simulink model "semi_GSTA_vgain"  (R2018b)
settings: Solver=FixedStepAuto  StartTime=0.0  StopTime=30  FixedStep=0.01  RelTol=1e-3
InitFcn:
  | parameters_semi_gsta_vgain
model workspace: external: MAT-File (data not in the file)
values from neighbouring files (symbols this model uses):
  sample_time = 0.05    [parameters_semi_gsta_const.m]    (also in parameters_semi_gsta_vgain.m)
  x = [1.07906107302 2.04168763414 1.85257539652 1.93323325754 2.1580260637 1.75776173681 1.89939965925 1.8937988199 1.84120163561 1.64161458182 1.95451206586 1.46429138729 ... (9600 elements, 1600x6)]    [dat_x.mat]    (also in parameters_semi_gsta_const.m = [300   300    0.3    0.3]; parameters_semi_gsta_vgain.m = [2   2   0.05     5      1    0.3    0.3  1   0.5])
  x0 = 0.5    [parameters_semi_gsta_const.m]    (also in parameters_semi_gsta_vgain.m)
undefined symbols (not defined in the file or in its folder): v0
libraries: sdolib x1
settings Model: Creator=DING  LastModifiedBy=DNN
settings SolverCC: ZeroCrossAlgorithm=Adaptive
settings OptimizationCC: DefaultParameterBehavior=Inlined  EnhancedBackFolding=on  PassReuseOutputArgsAs=Individual arguments  MaxStackSize=64  OptimizeBlockOrder=speed  DifferentSizesBufferReuse=on
settings DebuggingCC: IgnoredZcDiagnostic=none  ParameterTunabilityLossMsg=error
settings HardwareCC: ProdBitPerPointer=32  ProdBitPerSizeT=32  ProdBitPerPtrDiffT=32  ProdLargestAtomicInteger=Long  ProdLargestAtomicFloat=Double  ProdWordSize=32  ProdHWDeviceType=ARM Compatible->ARM 11
settings SFSimCC: MATLABDynamicMemAlloc=off
settings RTWCC: SystemTargetFile=ert.tlc  TemplateMakefile=ert_default_tmf  GenerateReport=on  Toolchain=Catkin  IncludeHyperlinkInReport=on  LaunchReport=on  GenerateTraceInfo=on  GenerateTraceReport=on  GenerateTraceReportSl=on  GenerateTraceReportSf=on  GenerateTraceReportEml=on
settings CodeAppCC: ForceParamTrailComments=on  IgnoreCustomStorageClasses=off  OperatorAnnotations=on  SimulinkDataObjDesc=on  SFDataObjDesc=on  InsertBlockDesc=on
settings ERTTargetCC: ERTCustomFileTemplate=example_file_process.tlc

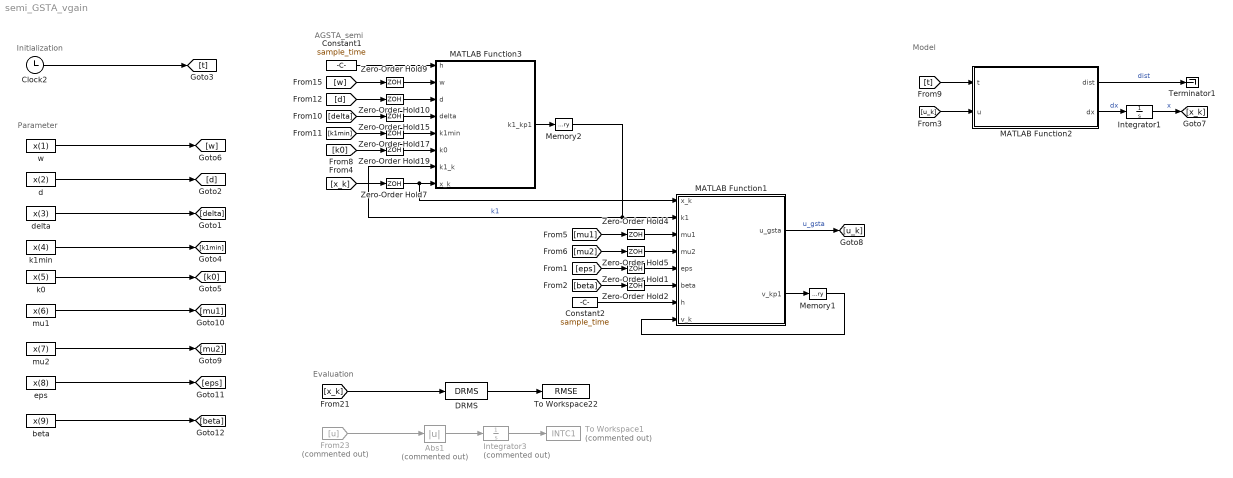
== system semi_GSTA_vgain ==
  note: Parameter
  note: Evaluation
  note: Initialization
  note: AGSTA_semi
  note: Model
  Abs1 : Abs  Commented=on
  Clock2 : Clock
  Constant1 : Constant  Value=sample_time  SampleTime=sample_time
  Constant2 : Constant  Value=sample_time  SampleTime=sample_time
  DRMS : sdolib/RMS Blocks/DRMS  Ts=sample_time
      settings: SourceProductBaseCode=SO
  From23 : From  Commented=on  GotoTag=u
  Integrator1 : Integrator  InitialCondition=x0
  Integrator3 : Integrator  Commented=on  InitialCondition=v0
  MATLAB Function1 : MATLAB Function  TreatAsAtomicUnit=on
  MATLAB Function2 : MATLAB Function  TreatAsAtomicUnit=on
  MATLAB Function3 : MATLAB Function  TreatAsAtomicUnit=on
  Memory1 : Memory  InheritSampleTime=on
  Memory2 : Memory  InheritSampleTime=on
  Terminator1 : Terminator
  To Workspace1 : ToWorkspace  Commented=on  VariableName=INTC1  SampleTime=-1
      settings: MaxDataPoints=1
  To Workspace22 : ToWorkspace  VariableName=RMSE  SampleTime=-1
      settings: MaxDataPoints=1
  Zero-Order Hold{1..2,4..5,7,9..10,15,17,19} (10 alike) : ZeroOrderHold  SampleTime=sample_time
  beta : Constant  Value=x(9)
  d : Constant  Value=x(2)
  delta : Constant  Value=x(3)
  eps : Constant  Value=x(8)
  k0 : Constant  Value=x(5)
  k1min : Constant  Value=x(4)
  mu1 : Constant  Value=x(6)
  mu2 : Constant  Value=x(7)
  w : Constant  Value=x(1)
  wires:
  Abs1/1 -> Integrator3/1
  d/1 -> [d]
  mu2/1 -> [mu2]
  From23/1 -> Abs1/1
  mu1/1 -> [mu1]
  Integrator3/1 -> To Workspace1/1
  Memory1/1 -> MATLAB Function1/8(v_k)
  [u_k] -> MATLAB Function2/2(u)
  [x_k] -> Zero-Order Hold7/1
  [mu1] -> Zero-Order Hold4/1
  Zero-Order Hold5/1 -> MATLAB Function1/4(mu2)
  DRMS/1 -> To Workspace22/1
  [mu2] -> Zero-Order Hold5/1
  MATLAB Function1/1(u_gsta) -> [u_k]  "u_gsta"
  Constant2/1 -> MATLAB Function1/7(h)
  MATLAB Function1/2(v_kp1) -> Memory1/1
  MATLAB Function2/2(dx) -> Integrator1/1  "dx"
  w/1 -> [w]
  Zero-Order Hold4/1 -> MATLAB Function1/3(mu1)
  [t] -> MATLAB Function2/1(t)
  Clock2/1 -> [t]
  Integrator1/1 -> [x_k]  "x"
  [x_k] -> DRMS/1
  MATLAB Function2/1(dist) -> Terminator1/1  "dist"
  [k0] -> Zero-Order Hold19/1
  Zero-Order Hold17/1 -> MATLAB Function3/5(k1min)
  Zero-Order Hold15/1 -> MATLAB Function3/4(delta)
  [w] -> Zero-Order Hold9/1
  [delta] -> Zero-Order Hold15/1
  [d] -> Zero-Order Hold10/1
  Zero-Order Hold19/1 -> MATLAB Function3/6(k0)
  MATLAB Function3/1(k1_kp1) -> Memory2/1
  Memory2/1 -> MATLAB Function3/7(k1_k), MATLAB Function1/2(k1)  "k1"
  Zero-Order Hold10/1 -> MATLAB Function3/3(d)
  [k1min] -> Zero-Order Hold17/1
  Zero-Order Hold9/1 -> MATLAB Function3/2(w)
  Zero-Order Hold7/1 -> MATLAB Function1/1(x_k), MATLAB Function3/8(x_k)
  delta/1 -> [delta]
  k1min/1 -> [k1min]
  k0/1 -> [k0]
  Constant1/1 -> MATLAB Function3/1(h)
  [beta] -> Zero-Order Hold2/1
  [eps] -> Zero-Order Hold1/1
  Zero-Order Hold1/1 -> MATLAB Function1/5(eps)
  Zero-Order Hold2/1 -> MATLAB Function1/6(beta)
  eps/1 -> [eps]
  beta/1 -> [beta]

== matlab function semi_GSTA_vgain/MATLAB Function1 ==
  data: x_k input; k1 input; mu1 input; mu2 input; eps input; beta input; h input; v_k input; u_gsta output; v_kp1 output
function [u_gsta, v_kp1] = GSTA(x_k, k1, mu1, mu2, eps, beta, h, v_k)

k2 = 2 * eps * k1 + beta + 4 * eps ^ 2;

lam_sum = - k1 * (mu1 * abs(x_k) ^ - 0.5 + mu2);
lam_multi = k2 * (0.5 * mu1 * abs(x_k) ^ - 1 + 1.5 * mu1 * mu2 * abs(x_k) ^ - 0.5 + mu2 ^ 2 );

if x_k == 0
        q_sum = 0;
        q_multi = 0;
else
        q_sum = (2 - h * lam_sum ) / (1 - h * lam_sum + h ^ 2 * lam_multi ); 
        q_multi = 1 / (1 - h * lam_sum + h ^ 2 * lam_multi );
end

u1_k = q_sum - 1;    % u1_k=q1+q2-1;
u2_k = 1 / h * (u1_k - q_multi);   % u2_k=1/h*(u1_k-q1*q2);


v_kp1 = v_k + u2_k * x_k;
u_gsta = 1 / h * ( - x_k + u1_k * x_k ) + v_kp1;

end

== matlab function semi_GSTA_vgain/MATLAB Function2 ==
  data: dist output; dx output; t input; u input
function [dist,dx]= Dynamic_Model(t,u)

% fx=0.6*sin(x)+0.7*x^2-1.5*x;
% dxt=0.8*cos(x)*x+0.05*cos(3*t)+0.08*sin(t);
% dx=fx+dxt+u;

dist=5*cos(t);
dx=u+dist;

end

== matlab function semi_GSTA_vgain/MATLAB Function3 ==
  data: h input; w input; d input; delta input; k1min input; k0 input; k1_k input; x_k input; k1_kp1 output
function k1_kp1= dk1(h, w, d, delta, k1min, k0,  k1_k, x_k)


if k1_k==0
     k1_kp1=k0;
elseif  k1_k<=k1min && abs(x_k)>delta
     k1_kp1=k1_k+h*w;
elseif  k1_k<=k1min && abs(x_k)<=delta
     k1_kp1=k1_k;
elseif  k1_k>k1min && abs(x_k)>delta
     k1_kp1=k1_k+h*w;
else
     k1_kp1=k1_k-h*d;
end 

end

% % % % % % % % % % % % % % % % 

% for i=1:6
% 
% if abs(s(i))<delta(i)
%     k1_kp1(i)=k1_k(i);
% else 
%     k1_kp1(i)=k1_k(i)+h*w(i);
% end
% 
% end

% if  abs(s(i))>delta(i)  
%         k1_kp1(i)=k1_k(i)+h*w(i);
% else
%        k1_kp1(i)=k1_k(i);
% end 


% if   k1_k(i)<=k1min(i) && abs(s(i))<=delta(i)
%         k1_kp1(i)=k1_k(i);
% elseif  k1_k(i)>k1min(i) && abs(s(i))>delta(i)
%         k1_kp1(i)=k1_k(i)-h*d(i);
% elseif  abs(s(i))>delta(i)  
%         k1_kp1(i)=k1_k(i)+h*w(i);
% else
%         k1_kp1(i)=0;
% end
% 
% end



% for i=1:6
% 
% if  k1_k(i)==0
%         k1_kp1(i)=k0(i);
% elseif   k1_k(i)<=k1min(i) && abs(s(i))<=delta(i)
%         k1_kp1(i)=k1_k(i);
% elseif  k1_k(i)>k1min(i) && abs(s(i))>delta(i)
%         k1_kp1(i)=k1_k(i)-h*d(i);
% else
%         k1_kp1(i)=k1_k(i)+h*w(i);
% end
% 
% end
% 
% end
